simulink model "gm_uz_pmsm_model_9ph_21b_all_double_vnl"  (R2021b)
settings: Solver=FixedStepAuto  StartTime=0.0  StopTime=0.8  RelTol=1e-3
PreLoadFcn:
  | uz_pmsm_model_9ph_init_parameter
undefined symbols (not defined in the file or in its folder): c, friction_coefficient, inertia, k_i_d, k_i_q, k_p_d, k_p_q, Kpd, L_d, L_o1, L_o2, L_q, L_x1, L_x2, L_y1, L_y2, L_zero, polepair, psi_pm, R_1, static_friction_torque, Tnd, ts
libraries: hdlmdlgenlib x124, dspsigops x19, simulink x16, slpidlib x2, spsAlphaBetaZerotodq0Lib x1, pid_lib x1, spsdq0toAlphaBetaZeroLib x1, hdlsllib x1
(part 4 of 4)

== system gm_uz_pmsm_model_9ph_21b_all_double_vnl/uz_pmsm_model_9ph/abc_to_dq/Line-Line to Phase voltage1/alpha_beta_0   to   abc ==
  "alpha, beta, 0  " : Inport  PortDimensions=3
  Gain4 : Gain  Gain="[ 1 0 1; -0.5   0.5*sqrt(3)  1; -0.5 -0.5*sqrt(3) 1 ]"  Multiplication=Matrix(K*u) (u vector)  ParamDataTypeStr=fixdt(1,18,16)  SaturateOnIntegerOverflow=on  OutDataTypeStr=Inherit: Same as input
  "a, b, c" : Outport
  wires:
  Gain4/1 -> "a, b, c"/1
  "alpha, beta, 0  "/1 -> Gain4/1

== system gm_uz_pmsm_model_9ph_21b_all_double_vnl/uz_pmsm_model_9ph/abc_to_dq/Line-Line to Phase voltage2/abc   to   alpha_beta_0 ==
  "a, b, c" : Inport  PortDimensions=3
  Gain2 : Gain  Gain=2/3  ParamDataTypeStr=fixdt(1,18,16)  SaturateOnIntegerOverflow=on  OutDataTypeStr=Inherit: Same as input
  Gain4 : Gain  Gain="[ 1   -0.5   -0.5; 0   0.5*sqrt(3)   -0.5*sqrt(3); 0.5  0.5  0.5 ]"  Multiplication=Matrix(K*u) (u vector)  ParamDataTypeStr=fixdt(1,18,16)  OutDataTypeStr=fixdt(1,25,12)  SaturateOnIntegerOverflow=on
  "alpha, beta, 0 " : Outport
  wires:
  Gain4/1 -> Gain2/1
  "a, b, c"/1 -> Gain4/1
  Gain2/1 -> "alpha, beta, 0 "/1

== system gm_uz_pmsm_model_9ph_21b_all_double_vnl/uz_pmsm_model_9ph/abc_to_dq/Line-Line to Phase voltage2/alpha_beta_0   to   abc ==
  "alpha, beta, 0  " : Inport  PortDimensions=3
  Gain4 : Gain  Gain="[ 1 0 1; -0.5   0.5*sqrt(3)  1; -0.5 -0.5*sqrt(3) 1 ]"  Multiplication=Matrix(K*u) (u vector)  ParamDataTypeStr=fixdt(1,18,16)  SaturateOnIntegerOverflow=on  OutDataTypeStr=Inherit: Same as input
  "a, b, c" : Outport
  wires:
  "alpha, beta, 0  "/1 -> Gain4/1
  Gain4/1 -> "a, b, c"/1

== system gm_uz_pmsm_model_9ph_21b_all_double_vnl/uz_pmsm_model_9ph/dq_model_9ph_vnl/mechanical_system/integrator ==
  in : Inport
  reset : Inport  Port=2
  Delay1 : Delay  DelayLength=1  ExternalReset=Level
      settings: InputPortMap=u0,r5
  Gain : Gain  Gain=ts  OutDataTypeStr=Inherit: Same as input
  Sum3 : Sum  Inputs=|++  OutDataTypeStr=Inherit: Same as first input
  outt : Outport
  wires:
  Sum3/1 -> Delay1/1
  Delay1/1 -> Sum3/2, outt/1
  in/1 -> Gain/1
  Gain/1 -> Sum3/1
  reset/1 -> Delay1/2

== system gm_uz_pmsm_model_9ph_21b_all_double_vnl/uz_pmsm_model_9ph/dq_model_9ph_vnl/pmsm/integrator ==
  in : Inport
  reset : Inport  Port=2
  Delay1 : Delay  DelayLength=1  ExternalReset=Level
      settings: InputPortMap=u0,r5
  Gain : Gain  Gain=ts  OutDataTypeStr=Inherit: Same as input
  Sum3 : Sum  Inputs=|++  OutDataTypeStr=Inherit: Same as first input
  outt : Outport
  wires:
  Sum3/1 -> Delay1/1
  Delay1/1 -> Sum3/2, outt/1
  in/1 -> Gain/1
  Gain/1 -> Sum3/1
  reset/1 -> Delay1/2

== system gm_uz_pmsm_model_9ph_21b_all_double_vnl/uz_pmsm_model_9ph/dq_model_9ph_vnl/pmsm/integrator1 ==
  in : Inport
  reset : Inport  Port=2
  Delay1 : Delay  DelayLength=1  ExternalReset=Level
      settings: InputPortMap=u0,r5
  Gain : Gain  Gain=ts  OutDataTypeStr=Inherit: Same as input
  Sum3 : Sum  Inputs=|++  OutDataTypeStr=Inherit: Same as first input
  outt : Outport
  wires:
  Sum3/1 -> Delay1/1
  Delay1/1 -> Sum3/2, outt/1
  in/1 -> Gain/1
  Gain/1 -> Sum3/1
  reset/1 -> Delay1/2

== system gm_uz_pmsm_model_9ph_21b_all_double_vnl/uz_pmsm_model_9ph/dq_model_9ph_vnl/pmsm/integrator2 ==
  in : Inport
  reset : Inport  Port=2
  Delay1 : Delay  DelayLength=1  ExternalReset=Level
      settings: InputPortMap=u0,r5
  Gain : Gain  Gain=ts  OutDataTypeStr=Inherit: Same as input
  Sum3 : Sum  Inputs=|++  OutDataTypeStr=Inherit: Same as first input
  outt : Outport
  wires:
  Sum3/1 -> Delay1/1
  Delay1/1 -> Sum3/2, outt/1
  in/1 -> Gain/1
  Gain/1 -> Sum3/1
  reset/1 -> Delay1/2

== system gm_uz_pmsm_model_9ph_21b_all_double_vnl/uz_pmsm_model_9ph/dq_model_9ph_vnl/pmsm/integrator3 ==
  in : Inport
  reset : Inport  Port=2
  Delay1 : Delay  DelayLength=1  ExternalReset=Level
      settings: InputPortMap=u0,r5
  Gain : Gain  Gain=ts  OutDataTypeStr=Inherit: Same as input
  Sum3 : Sum  Inputs=|++  OutDataTypeStr=Inherit: Same as first input
  outt : Outport
  wires:
  Sum3/1 -> Delay1/1
  Delay1/1 -> Sum3/2, outt/1
  in/1 -> Gain/1
  Gain/1 -> Sum3/1
  reset/1 -> Delay1/2

== system gm_uz_pmsm_model_9ph_21b_all_double_vnl/uz_pmsm_model_9ph/dq_model_9ph_vnl/pmsm/integrator4 ==
  in : Inport
  reset : Inport  Port=2
  Delay1 : Delay  DelayLength=1  ExternalReset=Level
      settings: InputPortMap=u0,r5
  Gain : Gain  Gain=ts  OutDataTypeStr=Inherit: Same as input
  Sum3 : Sum  Inputs=|++  OutDataTypeStr=Inherit: Same as first input
  outt : Outport
  wires:
  Sum3/1 -> Delay1/1
  Delay1/1 -> Sum3/2, outt/1
  in/1 -> Gain/1
  Gain/1 -> Sum3/1
  reset/1 -> Delay1/2

== system gm_uz_pmsm_model_9ph_21b_all_double_vnl/uz_pmsm_model_9ph/dq_model_9ph_vnl/pmsm/integrator5 ==
  in : Inport
  reset : Inport  Port=2
  Delay1 : Delay  DelayLength=1  ExternalReset=Level
      settings: InputPortMap=u0,r5
  Gain : Gain  Gain=ts  OutDataTypeStr=Inherit: Same as input
  Sum3 : Sum  Inputs=|++  OutDataTypeStr=Inherit: Same as first input
  outt : Outport
  wires:
  Sum3/1 -> Delay1/1
  Delay1/1 -> Sum3/2, outt/1
  in/1 -> Gain/1
  Gain/1 -> Sum3/1
  reset/1 -> Delay1/2

== system gm_uz_pmsm_model_9ph_21b_all_double_vnl/uz_pmsm_model_9ph/dq_model_9ph_vnl/pmsm/integrator6 ==
  in : Inport
  reset : Inport  Port=2
  Delay1 : Delay  DelayLength=1  ExternalReset=Level
      settings: InputPortMap=u0,r5
  Gain : Gain  Gain=ts  OutDataTypeStr=Inherit: Same as input
  Sum3 : Sum  Inputs=|++  OutDataTypeStr=Inherit: Same as first input
  outt : Outport
  wires:
  Sum3/1 -> Delay1/1
  Delay1/1 -> Sum3/2, outt/1
  in/1 -> Gain/1
  Gain/1 -> Sum3/1
  reset/1 -> Delay1/2

== system gm_uz_pmsm_model_9ph_21b_all_double_vnl/uz_pmsm_model_9ph/dq_model_9ph_vnl/pmsm/integrator7 ==
  in : Inport
  reset : Inport  Port=2
  Delay1 : Delay  DelayLength=1  ExternalReset=Level
      settings: InputPortMap=u0,r5
  Gain : Gain  Gain=ts  OutDataTypeStr=Inherit: Same as input
  Sum3 : Sum  Inputs=|++  OutDataTypeStr=Inherit: Same as first input
  outt : Outport
  wires:
  Sum3/1 -> Delay1/1
  Delay1/1 -> Sum3/2, outt/1
  in/1 -> Gain/1
  Gain/1 -> Sum3/1
  reset/1 -> Delay1/2

== system gm_uz_pmsm_model_9ph_21b_all_double_vnl/uz_pmsm_model_9ph/dq_model_9ph_vnl/pmsm/integrator8 ==
  in : Inport
  reset : Inport  Port=2
  Delay1 : Delay  DelayLength=1  ExternalReset=Level
      settings: InputPortMap=u0,r5
  Gain : Gain  Gain=ts  OutDataTypeStr=Inherit: Same as input
  Sum3 : Sum  Inputs=|++  OutDataTypeStr=Inherit: Same as first input
  outt : Outport
  wires:
  Sum3/1 -> Delay1/1
  Delay1/1 -> Sum3/2, outt/1
  in/1 -> Gain/1
  Gain/1 -> Sum3/1
  reset/1 -> Delay1/2

== matlab function gm_uz_pmsm_model_9ph_21b_all_double_vnl/uz_pmsm_model_9ph/Compare/Assert_M_Mi_axi/RelErrCheck/RelativeErrorCheck  ==
  data: P input; y output; R input; ToleranceValue parameter double
% Check if the relative error of R with respect to P is below
% ToleranceValue
% P, R are floating-point
function y = relErrCheck(P,R, ToleranceValue)
    tol = ToleranceValue;
    sz = numel(P);
    assert(sz == numel(R), 'Inputs P and R have different sizes.');
    y = false(1, sz);

    for ii=1:sz
        if (isnan(P(ii)) || isnan(R(ii)))
            if (isnan(P(ii)) && isnan(R(ii)))
                y(ii) = true;
            end
        elseif (isinf(P(ii)) || isinf(R(ii)))
            y(ii) = (P(ii) == R(ii));
        elseif (P(ii) == 0)
            y(ii) = (R(ii) == 0);
        else
            absdiff = abs(P(ii) - R(ii));
            relerr = absdiff/abs(P(ii));
            y(ii) = (relerr <= tol);
        end
    end
end

== matlab function gm_uz_pmsm_model_9ph_21b_all_double_vnl/uz_pmsm_model_9ph/Compare/Assert_omega_out_axi/RelErrCheck/RelativeErrorCheck  ==
  data: P input; y output; R input; ToleranceValue parameter double
% Check if the relative error of R with respect to P is below
% ToleranceValue
% P, R are floating-point
function y = relErrCheck(P,R, ToleranceValue)
    tol = ToleranceValue;
    sz = numel(P);
    assert(sz == numel(R), 'Inputs P and R have different sizes.');
    y = false(1, sz);

    for ii=1:sz
        if (isnan(P(ii)) || isnan(R(ii)))
            if (isnan(P(ii)) && isnan(R(ii)))
                y(ii) = true;
            end
        elseif (isinf(P(ii)) || isinf(R(ii)))
            y(ii) = (P(ii) == R(ii));
        elseif (P(ii) == 0)
            y(ii) = (R(ii) == 0);
        else
            absdiff = abs(P(ii) - R(ii));
            relerr = absdiff/abs(P(ii));
            y(ii) = (relerr <= tol);
        end
    end
end

== matlab function gm_uz_pmsm_model_9ph_21b_all_double_vnl/uz_pmsm_model_9ph/Compare/Assert_voltage_input_dq_axi_fb/RelErrCheck/RelativeErrorCheck  ==
  data: P input; y output; R input; ToleranceValue parameter double
% Check if the relative error of R with respect to P is below
% ToleranceValue
% P, R are floating-point
function y = relErrCheck(P,R, ToleranceValue)
    tol = ToleranceValue;
    sz = numel(P);
    assert(sz == numel(R), 'Inputs P and R have different sizes.');
    y = false(1, sz);

    for ii=1:sz
        if (isnan(P(ii)) || isnan(R(ii)))
            if (isnan(P(ii)) && isnan(R(ii)))
                y(ii) = true;
            end
        elseif (isinf(P(ii)) || isinf(R(ii)))
            y(ii) = (P(ii) == R(ii));
        elseif (P(ii) == 0)
            y(ii) = (R(ii) == 0);
        else
            absdiff = abs(P(ii) - R(ii));
            relerr = absdiff/abs(P(ii));
            y(ii) = (relerr <= tol);
        end
    end
end

== matlab function gm_uz_pmsm_model_9ph_21b_all_double_vnl/uz_pmsm_model_9ph/Compare/Assert_currents_dq_output_axi/RelErrCheck/RelativeErrorCheck  ==
  data: P input; y output; R input; ToleranceValue parameter double
% Check if the relative error of R with respect to P is below
% ToleranceValue
% P, R are floating-point
function y = relErrCheck(P,R, ToleranceValue)
    tol = ToleranceValue;
    sz = numel(P);
    assert(sz == numel(R), 'Inputs P and R have different sizes.');
    y = false(1, sz);

    for ii=1:sz
        if (isnan(P(ii)) || isnan(R(ii)))
            if (isnan(P(ii)) && isnan(R(ii)))
                y(ii) = true;
            end
        elseif (isinf(P(ii)) || isinf(R(ii)))
            y(ii) = (P(ii) == R(ii));
        elseif (P(ii) == 0)
            y(ii) = (R(ii) == 0);
        else
            absdiff = abs(P(ii) - R(ii));
            relerr = absdiff/abs(P(ii));
            y(ii) = (relerr <= tol);
        end
    end
end

== matlab function gm_uz_pmsm_model_9ph_21b_all_double_vnl/uz_pmsm_model_9ph/Compare/Assert_theta_el_axi/RelErrCheck/RelativeErrorCheck  ==
  data: P input; y output; R input; ToleranceValue parameter double
% Check if the relative error of R with respect to P is below
% ToleranceValue
% P, R are floating-point
function y = relErrCheck(P,R, ToleranceValue)
    tol = ToleranceValue;
    sz = numel(P);
    assert(sz == numel(R), 'Inputs P and R have different sizes.');
    y = false(1, sz);

    for ii=1:sz
        if (isnan(P(ii)) || isnan(R(ii)))
            if (isnan(P(ii)) && isnan(R(ii)))
                y(ii) = true;
            end
        elseif (isinf(P(ii)) || isinf(R(ii)))
            y(ii) = (P(ii) == R(ii));
        elseif (P(ii) == 0)
            y(ii) = (R(ii) == 0);
        else
            absdiff = abs(P(ii) - R(ii));
            relerr = absdiff/abs(P(ii));
            y(ii) = (relerr <= tol);
        end
    end
end
